simulink model "OL_model"  (R2024b)
settings: Solver=VariableStepAuto  StartTime=0.0  StopTime=10.0  RelTol=1e-3
undefined symbols (not defined in the file or in its folder): para
settings Model: Creator=feder  LastModifiedBy=feder

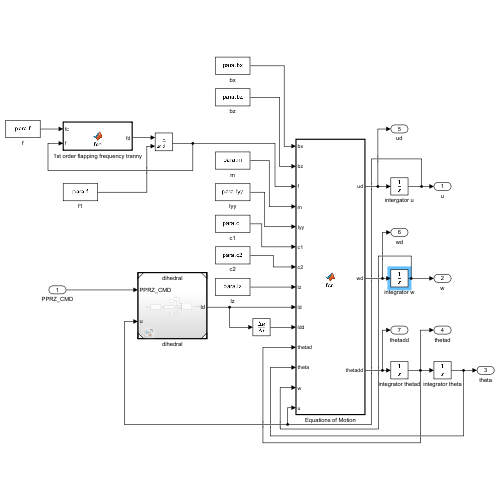
[thumbnail: Simulink's stored preview of the top-level diagram]
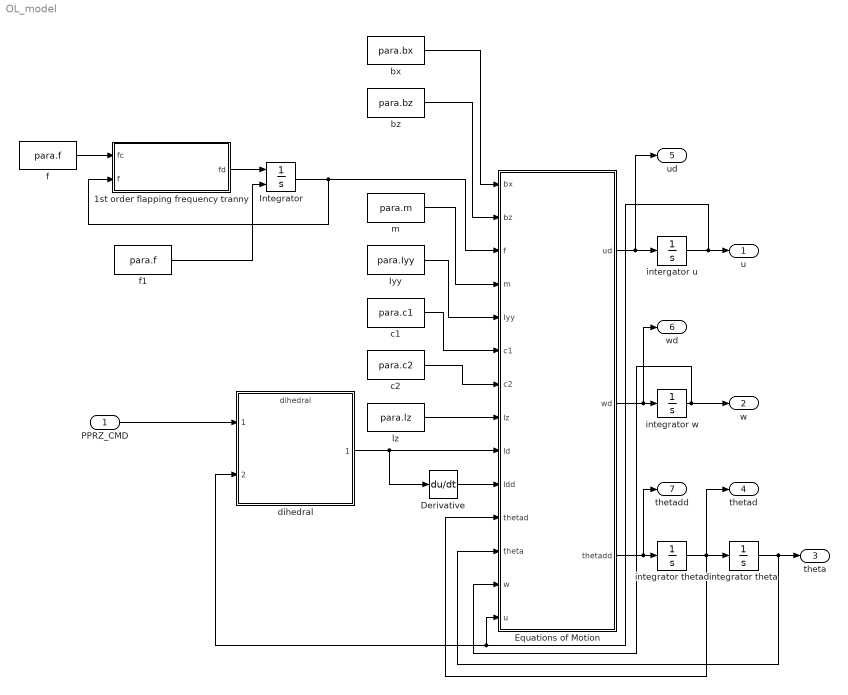
== system OL_model ==
  PPRZ_CMD : Inport
  1st order flapping frequency tranny : MATLAB Function  TreatAsAtomicUnit=on
  Derivative : Derivative
  Equations of Motion : MATLAB Function  TreatAsAtomicUnit=on
  Integrator : Integrator  InitialConditionSource=external
  Iyy : Constant  Value=para.Iyy
  bx : Constant  Value=para.bx
  bz : Constant  Value=para.bz
  c1 : Constant  Value=para.c1  VectorParams1D=off
  c2 : Constant  Value=para.c2
  dihedral : ModelReference  ModelNameDialog=dihedral.slx  SimulationMode=Normal  ModelReferenceVersion=1.18
  f : Constant  Value=para.f
  f1 : Constant  Value=para.f
  integrator theta : Integrator
  integrator thetad : Integrator
  integrator w : Integrator  InitialCondition=para.w0
  intergator u : Integrator
  lz : Constant  Value=para.lz
  m : Constant  Value=para.m
  u : Outport
  w : Outport  Port=2
  theta : Outport  Port=3
  thetad : Outport  Port=4
  ud : Outport  Port=5
  wd : Outport  Port=6
  thetadd : Outport  Port=7
  wires:
  PPRZ_CMD/1 -> dihedral/1
  dihedral/1 -> Equations of Motion/9(ld), Derivative/1
  Derivative/1 -> Equations of Motion/10(ldd)
  Equations of Motion/1(ud) -> intergator u/1, ud/1
  Equations of Motion/2(wd) -> wd/1, integrator w/1
  integrator w/1 -> Equations of Motion/13(w), w/1
  intergator u/1 -> u/1, Equations of Motion/14(u), dihedral/2
  Equations of Motion/3(thetadd) -> thetadd/1, integrator thetad/1
  integrator thetad/1 -> integrator theta/1, Equations of Motion/11(thetad), thetad/1
  integrator theta/1 -> Equations of Motion/12(theta), theta/1
  bx/1 -> Equations of Motion/1(bx)
  lz/1 -> Equations of Motion/8(lz)
  bz/1 -> Equations of Motion/2(bz)
  m/1 -> Equations of Motion/4(m)
  Iyy/1 -> Equations of Motion/5(Iyy)
  c1/1 -> Equations of Motion/6(c1)
  c2/1 -> Equations of Motion/7(c2)
  f/1 -> 1st order flapping frequency tranny/1(fc)
  1st order flapping frequency tranny/1(fd) -> Integrator/1
  f1/1 -> Integrator/2
  Integrator/1 -> 1st order flapping frequency tranny/2(f), Equations of Motion/3(f)

== matlab function OL_model/Equations of Motion ==
  data: bx input; bz input; f input; m input; Iyy input; c1 input; c2 input; lz input; ld input; ldd input; thetad input; theta input; ud output; wd output; thetadd output; w input; u input
function [ud, wd, thetadd] = fcn(bx, bz, f, m, Iyy, c1, c2, lz, ld, ldd,  thetad, theta, w, u)
g = 9.81;
ud = thetad*w*0 + g*sin(theta) - 2*(bx / m)*(u + lz*thetad - ldd);

T = 2*(c1*f+c2);

wd = -thetad*u*0 + g*cos(theta) - T/m - 2*(bz/m)*(w + ld*thetad);

thetadd = (1/Iyy)*(-2*bx*lz*(-u + lz*thetad + ldd) + 2*bz*ld*(- w - ld*thetad) - T*ld);

%% As in paper

% g = 9.81;
% ud = -thetad*w*0 - g*sin(theta) - 2*(bx / m)*(u - lz*thetad + ldd);

% T = 2*(c1*f+c2);

% wd = thetad*u*0 + g*cos(theta) - T/m - 2*(bz/m)*(w - ld*thetad);

% thetadd = (1/Iyy)*(2*-bx*lz*(u - lz*thetad - ldd) + 2*bz*ld*(w - ld*thetad) - T*ld);


%% His model
% ud = -sin(theta)*g - 2*bx/m*u + lz*2*bx*thetad/m + 2*bx*lpd/m;
% 

% wd = cos(theta)*g - 2*(c1*f + c2)/m - 2*bz*w/m - 2*bz*(lp)*thetad/m;  
% 
% thetadd = (2*bx*lz*u - 2*bx*lz^2*(thetad) - 2*bx*lz*(lpd)...
% - 2*c1*f.*(lp+lx) - 2*c2*(lp) - 2*bz*w.*(lp) - 2*bz*(lp).^2.*(thetad))/Iyy;
end

== matlab function OL_model/1st order flapping frequency tranny ==
  data: fc input; fd output; f input
function fd = fcn(fc,f)

% fd = 11.04*fc - 12.56*f;
fd = 12.56*fc - 12.56*f;
